simulink model "vipstabilize"  (R2015b)
settings: Solver=FixedStepDiscrete  StartTime=0.0  StopTime=inf  RelTol=1e-3
undefined symbols (not defined in the file or in its folder): gray
libraries: visiontextngfix x3, visiongeotforms x2, visionsinks x2, dspvision x1, vipmisc x1, visionanalysis x1
Description:
  | Image stabilization demo.
settings Model: Tag="0  0  0  0  0  1"  FPTRunName=Active  ExtModeAutoUpdateStatusClock=off  Creator=The MathWorks, Inc.  LastModifiedBy=The MathWorks, Inc.
settings DataIOCC: SaveFormat=Array  SaveOutput=off  SaveTime=off  SignalLoggingName=logsOut
settings OptimizationCC: ExpressionDepthLimit=2147483647  InitFltsAndDblsToZero=on  BufferReusableBoundary=off
settings DebuggingCC: UnderspecifiedInitializationDetection=Classic  MergeDetectMultiDrivingBlocksExec=none  CheckExecutionContextPreStartOutputMsg=on  CheckExecutionContextRuntimeOutputMsg=on  SignalResolutionControl=TryResolveAllWithWarning  InheritedTsInSrcMsg=none  MultiTaskDSMMsg=warning  MultiTaskCondExecSysMsg=none  FcnCallInpInsideContextMsg=UseLocalSettings  BusObjectLabelMismatch=none  StateNameClashWarn=warning  StrictBusMsg=None
settings HardwareCC: ProdBitPerPointer=32  ProdLargestAtomicFloat=None  ProdIntDivRoundTo=Undefined  ProdEndianess=Unspecified  ProdWordSize=32  ProdHWDeviceType=Specified  TargetBitPerLong=64  TargetBitPerPointer=64  TargetLongLongMode=on  TargetIntDivRoundTo=Zero  TargetEndianess=LittleEndian  TargetWordSize=64  TargetHWDeviceType=Generic->MATLAB Host Computer  ProdEqTarget=off
settings ModelReferenceCC: UpdateModelReferenceTargets=IfOutOfDate
settings GRTTargetCC: TargetFcnLib=ansi_tfl_tmw_new.mat  GeneratePreprocessorConditionals=Disable all  CombineOutputUpdateFcns=off  GRTInterface=on
settings ConfigComp: CovModelRefEnable=Off

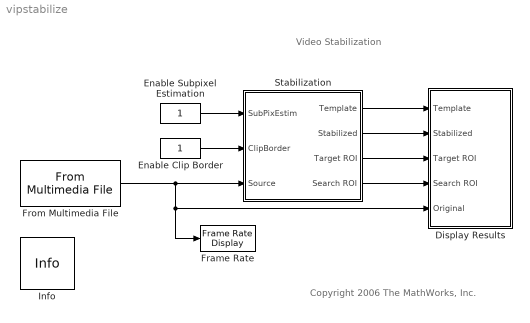
== system vipstabilize ==
  note: Video Stabilization
  note: Copyright 2006 The MathWorks, Inc.
  Display Results : Subsystem
  Enable Clip Border : Constant  VectorParams1D=off  OutDataTypeStr=boolean
  Enable Subpixel Estimation : Constant  VectorParams1D=off  OutDataTypeStr=boolean
  Frame Rate : visionsinks/Frame Rate Display  UpdateRate=10
  From Multimedia File : dspvision/From Multimedia File  inputFilename=shaky_car.avi  loop=on  numPlays=inf  outputStreams=Video only  videoDataType=single  audioDataType=int16  inheritSampleTime=on  userDefinedSampleTime=1/30  noAudioOutput=off  isIntensityVideo=off  fourcc=Intensity  colorVideoFormat=Separate color signals  outputEOF=off  dataOrg=Column-major  audioFrameSize=1024  computeAudioFrameSize=off  outSamplingMode=Frame based
  Info : vipmisc/Info  SystemSampleTime=-1
  Stabilization : Subsystem  mask(Stabilization){template_orig=[109 100], template_size=[18 22], search_border=[10 15]}
      mask prompts: template_orig "Upper left corner of the template [x y]:"; template_size "Template size [height width]:"; search_border "Search border [num_rows num_cols]:"
      mask help:
      | Remove motion from the input video signal.
      |
      | Use Upper left corner of template and Template size parameters to define the location and size of the target on the first frame of the input video.  Use Search border to define size of the search region around the target.
      |
      | Note:  You can right-click on Stabilization subsystem and select "Look Under Mask" to explore the design of the underlying algorithm.
      mask init:
      | pos.template_orig = fliplr(template_orig); % Use R,C internally
      | pos.template_size = template_size;
      | pos.search_border = search_border;
      | pos.template_center = floor((template_size-1)/2);
      | pos.template_center_pos = pos.template_orig + ...
      |     pos.template_center - 1;
      mask Help: Demo subsystem in support of the Video Stabilization demo.  You can right-click on Stabilization subsystem and select "Look Under Mask" to explore the design of the underlying algorithm.
  wires:
  Stabilization/1(Template) -> Display Results/1(Template)
  From Multimedia File/1 -> Display Results/5(Original), Frame Rate/1, Stabilization/3(Source)
  Stabilization/2(Stabilized) -> Display Results/2(Stabilized)
  Enable Subpixel Estimation/1 -> Stabilization/1(SubPixEstim)
  Stabilization/3(Target ROI) -> Display Results/3(Target ROI)
  Stabilization/4(Search ROI) -> Display Results/4(Search ROI)
  Enable Clip Border/1 -> Stabilization/2(ClipBorder)

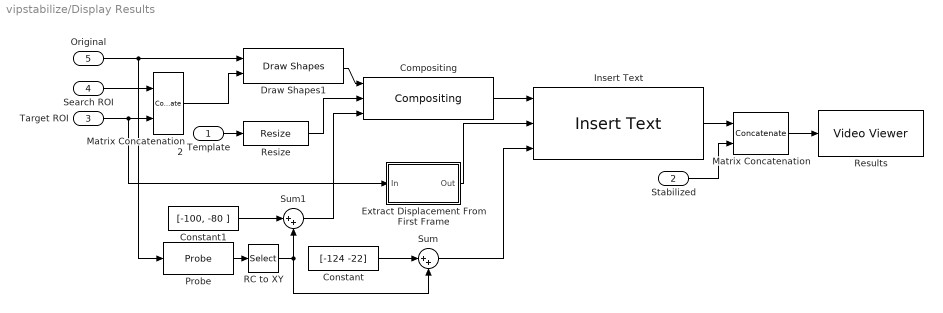
== system vipstabilize/Display Results ==
  Template : Inport
  Stabilized : Inport  Port=2
  Target ROI : Inport  Port=3
  Search ROI : Inport  Port=4
  Original : Inport  Port=5
  Compositing : visiontextngfix/Compositing  operation=Binary mask  bFacSrc=Specify via dialog  mFacSrc=Specify via dialog  bFactor=1  mFactor=1  source=Input port  coordinates=[160 220]  prodOutputMode=Binary point scaling  prodOutputWordLength=32  prodOutputFracLength=10  roundingMode=Floor  overflowMode=off
  Constant : Constant  Value=[-124 -22]
  Constant1 : Constant  Value=[-100, -80 ]
  Draw Shapes1 : visiontextngfix/Draw Shapes  shape=Rectangles  fill=off  lineWidth=1  fillClrSource=Specify via dialog  display=White  intensity=200  color=[200 255 100]  opacity=0.6  viewport=Entire image  antialiasing=off  inType=Intensity  imagePorts=One multidimensional signal  prodOutputMode=Binary point scaling  prodOutputWordLength=32  prodOutputFracLength=14  memoryMode=Specify word length  memoryWordLength=16  memoryFracLength=15  roundingMode=Floor  overflowMode=off
  Extract Displacement From First Frame : Subsystem
  Insert Text : visiontextngfix/Insert Text  inputType=Obsolete  theText='(%+05.1f,%+05.1f)'  getTextLocFrom=Input port  textLoc=[218 196]  getTextColorFrom=Specify via dialog  textColor=1  getTextIntensityFrom=Specify via dialog  textIntensity=1  getTextOpacityFrom=Specify via dialog  textOpacity=1.0  dummyVar2=0  dummyVar3=0  dummyVar4=0  imagePorts=One multidimensional signal  isInputTransposed=off  fontFace=LucidaTypewriterRegular  dummyVar1=0  blockFontSize=14  antiAliased=on
  Matrix Concatenation : Concatenate  Mode=Multidimensional array  ConcatenateDimension=2
  Matrix Concatenation2 : Concatenate  Mode=Multidimensional array
  Probe : Probe  ProbeWidth=off  ProbeSampleTime=off  ProbeComplexSignal=off  ProbeSignalDimensions=on
  RC to XY : Selector  IndexOptions=Index vector (dialog)  Indices=[2 1]  OutputSizes=1
  Resize : visiongeotforms/Resize  specify=Output size as a percentage of input size  rfactor=300  outCols=25  outRows=25  outRowsCols=[25 35]  interp_method=Bilinear  antialias=on  useROI=off  roiFlag=off  prodOutputMode=Binary point scaling  prodOutputWordLength=32  prodOutputFracLength=10  roundingMode=Nearest  overflowMode=on
  Results : visionsinks/Video Viewer  inputType=Obsolete7b  imagePorts=One multidimensional signal  useColorMap=off  colormapValue=gray(256)  specRange=off  minInputVal=0  maxInputVal=255  FigPos=[83 372 640 262]  AxisZoom=on  trueSizedOnce=on  OpenAtMdlStart=on  DefaultConfigurationName=vipscopes.VideoViewerScopeCfg
  Sum : Sum  Inputs=|++
  Sum1 : Sum  Inputs=|++
  wires:
  Stabilized/1 -> Matrix Concatenation/2
  Extract Displacement From First Frame/1(Out) -> Insert Text/2
  Draw Shapes1/1 -> Compositing/1
  Matrix Concatenation2/1 -> Draw Shapes1/2
  Search ROI/1 -> Matrix Concatenation2/1
  Target ROI/1 -> Matrix Concatenation2/2, Extract Displacement From First Frame/1(In)
  Original/1 -> Draw Shapes1/1, Probe/1
  Matrix Concatenation/1 -> Results/1
  Compositing/1 -> Insert Text/1
  Insert Text/1 -> Matrix Concatenation/1
  Resize/1 -> Compositing/2
  Constant1/1 -> Sum1/1
  Sum1/1 -> Compositing/3
  Probe/1 -> RC to XY/1
  Sum/1 -> Insert Text/3
  Constant/1 -> Sum/1
  Template/1 -> Resize/1
  RC to XY/1 -> Sum1/2, Sum/2

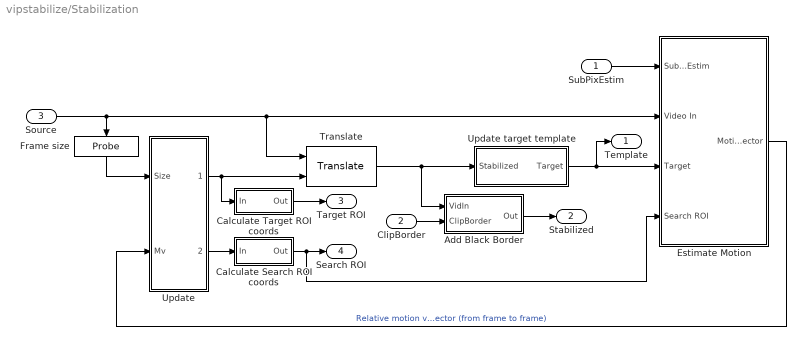
== system vipstabilize/Stabilization ==
  SubPixEstim : Inport
  ClipBorder : Inport  Port=2
  Source : Inport  Port=3
  Add Black Border : Subsystem
  Calculate Search ROI coords : Subsystem
  Calculate Target ROI coords : Subsystem
  Estimate Motion : Subsystem
  Frame size : Probe  ProbeWidth=off  ProbeSampleTime=off  ProbeComplexSignal=off  ProbeSignalDimensions=on  ProbeDimensionsDataType=Same as input
  Translate : visiongeotforms/Translate  outSizeT=Same as input image  src_trans=Input port  translation="[1.5  2.3]"  maxOffset=[8 10]  fillVal=0  interpMethod=Bilinear  firstCoeffMode=Binary point scaling  firstCoeffWordLength=16  firstCoeffFracLength=6  prodOutputMode=Binary point scaling  prodOutputWordLength=16  prodOutputFracLength=10  roundingMode=Floor  overflowMode=off
  Update : Subsystem
  Update target template : Subsystem
  Template : Outport
  Stabilized : Outport  Port=2
  Target ROI : Outport  Port=3
  Search ROI : Outport  Port=4
  wires:
  ClipBorder/1 -> Add Black Border/2(ClipBorder)
  Add Black Border/1(Out) -> Stabilized/1
  Calculate Search ROI coords/1(Out) -> Search ROI/1, Estimate Motion/4(Search ROI)
  Calculate Target ROI coords/1(Out) -> Target ROI/1
  SubPixEstim/1 -> Estimate Motion/1(SubPixEstim)
  Update/1(Offset) -> Calculate Target ROI coords/1(In), Translate/2
  Update/2(Location) -> Calculate Search ROI coords/1(In)
  Update target template/1(Target) -> Template/1, Estimate Motion/3(Target)
  Source/1 -> Translate/1, Estimate Motion/2(Video In), Frame size/1
  Translate/1 -> Add Black Border/1(VidIn), Update target template/1(Stabilized)
  Estimate Motion/1(Motion Vector) -> Update/2(Mv)  "Relative motion vector (from frame to frame)"
  Frame size/1 -> Update/1(Size)

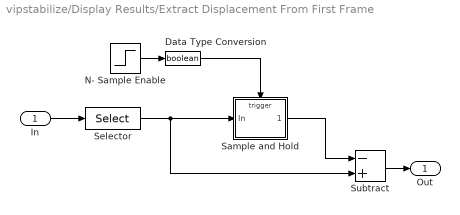
== system vipstabilize/Display Results/Extract Displacement From First Frame ==
  In : Inport
  Data Type Conversion : DataTypeConversion  OutDataTypeStr=boolean
  N- Sample Enable : Step  Time=0
  Sample and Hold : Subsystem  TreatAsAtomicUnit=on  mask{initCond=0}
      mask prompts: initCond "Initial Condition"
  Selector : Selector  NumberOfDimensions=2  InputPortWidth=3  IndexOptions=Index vector (dialog),Index vector (dialog)  Indices=1,[1 2]  OutputSizes=1,1
  Subtract : Sum  Inputs=-+
  Out : Outport
  wires:
  Data Type Conversion/1 -> Sample and Hold/Trigger
  In/1 -> Selector/1
  Selector/1 -> Subtract/2, Sample and Hold/1(In)
  Subtract/1 -> Out/1
  Sample and Hold/1(" ") -> Subtract/1
  N- Sample Enable/1 -> Data Type Conversion/1

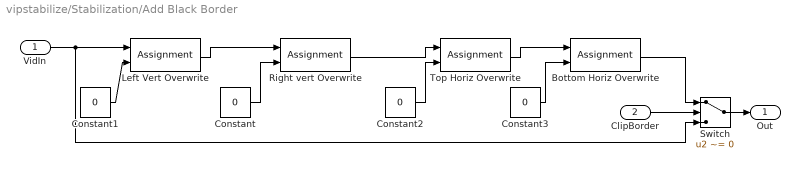
== system vipstabilize/Stabilization/Add Black Border ==
  VidIn : Inport
  ClipBorder : Inport  Port=2
  Bottom Horiz Overwrite : Assignment  NumberOfDimensions=2  IndexOptions=Index vector (dialog),Assign all  Indices=[240-(pos.search_border(2)+4):240],[320-(pos.search_border(2)+4):320]  OutputSizes=1,1
  Constant{,1..3} (4 alike) : Constant  Value=0  OutDataTypeStr=single
  Left Vert Overwrite : Assignment  NumberOfDimensions=2  IndexOptions=Assign all,Index vector (dialog)  Indices=1:end,1:(pos.search_border(2)+4)  OutputSizes=1,1
  Right vert Overwrite : Assignment  NumberOfDimensions=2  IndexOptions=Assign all,Index vector (dialog)  Indices=1:end,[320-(pos.search_border(2)+4):320]  OutputSizes=1,1
  Switch : Switch  Criteria=u2 ~= 0  ZeroCross=off
  Top Horiz Overwrite : Assignment  NumberOfDimensions=2  IndexOptions=Index vector (dialog),Assign all  Indices=[1:pos.search_border(1)+4],[320-(pos.search_border(2)+4):320]  OutputSizes=1,1
  Out : Outport
  wires:
  VidIn/1 -> Switch/3, Left Vert Overwrite/1
  Left Vert Overwrite/1 -> Right vert Overwrite/1
  Right vert Overwrite/1 -> Top Horiz Overwrite/1
  Top Horiz Overwrite/1 -> Bottom Horiz Overwrite/1
  ClipBorder/1 -> Switch/2
  Bottom Horiz Overwrite/1 -> Switch/1
  Switch/1 -> Out/1
  Constant/1 -> Right vert Overwrite/2
  Constant1/1 -> Left Vert Overwrite/2
  Constant2/1 -> Top Horiz Overwrite/2
  Constant3/1 -> Bottom Horiz Overwrite/2

== system vipstabilize/Stabilization/Calculate Search ROI coords ==
  In : Inport
  Constant : Constant  Value=fliplr(pos.template_size + 2*pos.search_border)  VectorParams1D=off  OutDataTypeStr=single
  Flip : Selector  NumberOfDimensions=2  IndexOptions=Index vector (dialog),Index vector (dialog)  Indices=1,[2 1]  OutputSizes=1,1
  Matrix Concatenation : Concatenate  Mode=Multidimensional array  ConcatenateDimension=2
  Out : Outport
  wires:
  Matrix Concatenation/1 -> Out/1
  In/1 -> Flip/1
  Constant/1 -> Matrix Concatenation/2
  Flip/1 -> Matrix Concatenation/1

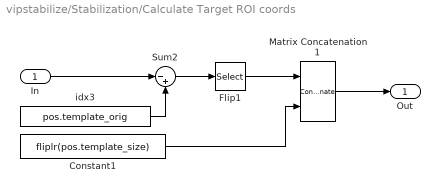
== system vipstabilize/Stabilization/Calculate Target ROI coords ==
  In : Inport
  Constant1 : Constant  Value=fliplr(pos.template_size)  VectorParams1D=off  OutDataTypeStr=single
  Flip1 : Selector  NumberOfDimensions=2  IndexOptions=Index vector (dialog),Index vector (dialog)  Indices=1,[2 1]  OutputSizes=1,1
  Matrix Concatenation1 : Concatenate  Mode=Multidimensional array  ConcatenateDimension=2
  Sum2 : Sum  Inputs=|-+
  idx3 : Constant  Value=pos.template_orig  VectorParams1D=off  OutDataTypeStr=single
  Out : Outport
  wires:
  Matrix Concatenation1/1 -> Out/1
  idx3/1 -> Sum2/2
  Sum2/1 -> Flip1/1
  Constant1/1 -> Matrix Concatenation1/2
  Flip1/1 -> Matrix Concatenation1/1
  In/1 -> Sum2/1

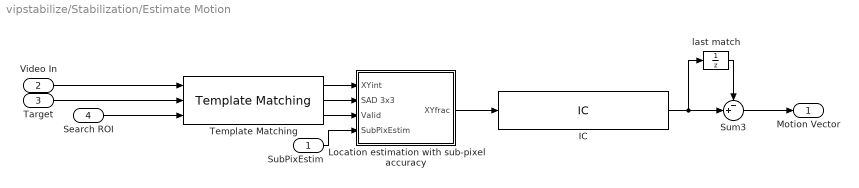
== system vipstabilize/Stabilization/Estimate Motion ==
  SubPixEstim : Inport
  Video In : Inport  Port=2
  Target : Inport  Port=3
  Search ROI : Inport  Port=4
  IC : InitialCondition  Value=fliplr(pos.template_center_pos)
  Location estimation with sub-pixel accuracy : Subsystem
  Sum3 : Sum  Inputs=-+|
  Template Matching : visionanalysis/Template Matching  metric=Sum of absolute differences  output=Best match location  method=Exhaustive  nMetric=on  nSize=3  roi=on  roiValid=off  accumMode=Binary point scaling  accumWordLength=32  accumFracLength=0  prodOutputMode=Binary point scaling  prodOutputWordLength=32  prodOutputFracLength=0  roundingMode=Floor  overflowMode=off
  last match : UnitDelay  InitialCondition=fliplr(pos.template_center_pos)  SampleTime=-1
  Motion Vector : Outport
  wires:
  IC/1 -> last match/1, Sum3/2
  last match/1 -> Sum3/1
  Location estimation with sub-pixel accuracy/1(XYfrac) -> IC/1
  SubPixEstim/1 -> Location estimation with sub-pixel accuracy/4(SubPixEstim)
  Search ROI/1 -> Template Matching/3
  Sum3/1 -> Motion Vector/1
  Target/1 -> Template Matching/2
  Template Matching/1 -> Location estimation with sub-pixel accuracy/1(XYint)
  Template Matching/2 -> Location estimation with sub-pixel accuracy/2(SAD 3x3)
  Template Matching/3 -> Location estimation with sub-pixel accuracy/3(Valid)
  Video In/1 -> Template Matching/1

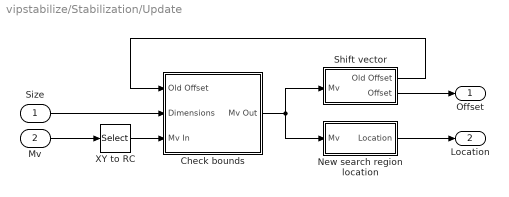
== system vipstabilize/Stabilization/Update ==
  Size : Inport
  Mv : Inport  Port=2
  Check bounds : Subsystem
  New search region location : Subsystem
  Shift vector : Subsystem
  XY to RC : Selector  NumberOfDimensions=2  IndexOptions=Index vector (dialog),Index vector (dialog)  Indices=1,[2 1]  OutputSizes=1,1
  Offset : Outport
  Location : Outport  Port=2
  wires:
  Shift vector/1(Old Offset) -> Check bounds/1(Old Offset)
  Mv/1 -> XY to RC/1
  New search region location/1(Location) -> Location/1
  Shift vector/2(Offset) -> Offset/1
  Size/1 -> Check bounds/2(Dimensions)
  Check bounds/1(Mv Out) -> Shift vector/1(Mv), New search region location/1(Mv)
  XY to RC/1 -> Check bounds/3(Mv In)

== system vipstabilize/Stabilization/Update target template ==
  note: cut out new template
  Stabilized : Inport
  Delay : UnitDelay  SampleTime=-1
  Selector : Selector  NumberOfDimensions=2  InputPortWidth=3  IndexOptions=Index vector (dialog),Index vector (dialog)  Indices=pos.template_orig(1)-1 : pos.template_orig(1)+pos.template_size(1)-2,pos.template_orig(2)-1 : pos.template_orig(2)+pos.template_size(2)-2  OutputSizes=1,1
  Target : Outport
  wires:
  Delay/1 -> Target/1
  Stabilized/1 -> Selector/1
  Selector/1 -> Delay/1

== system vipstabilize/Display Results/Extract Displacement From First Frame/Sample and Hold ==
  In : Inport
  Trigger : TriggerPort  ZeroCross=off
  " " : Outport  InitialOutput=initCond
  wires:
  In/1 -> " "/1

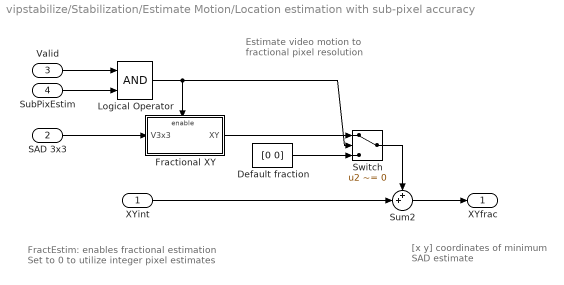
== system vipstabilize/Stabilization/Estimate Motion/Location estimation with sub-pixel accuracy ==
  note: [x y] coordinates of
      | minimum SAD estimate
  note: FractEstim: enables fractional estimation
      | Set to 0 to utilize integer pixel estimates
  note: Estimate video motion to
      | fractional pixel resolution
  XYint : Inport
  SAD 3x3 : Inport  Port=2
  Valid : Inport  Port=3
  SubPixEstim : Inport  Port=4
  Default fraction : Constant  Value=[0 0]  VectorParams1D=off  OutDataTypeStr=Inherit: Inherit via back propagation
  Fractional XY : Subsystem
  Logical Operator : Logic  AllPortsSameDT=off  OutDataTypeStr=boolean
  Sum2 : Sum  Inputs=++|  OutDataTypeStr=single
  Switch : Switch  Criteria=u2 ~= 0
  XYfrac : Outport
  wires:
  SubPixEstim/1 -> Logical Operator/2
  XYint/1 -> Sum2/2
  Fractional XY/1(XY) -> Switch/1
  Switch/1 -> Sum2/1
  Default fraction/1 -> Switch/3
  Sum2/1 -> XYfrac/1
  SAD 3x3/1 -> Fractional XY/1(V3x3)
  Logical Operator/1 -> Fractional XY/Enable, Switch/2
  Valid/1 -> Logical Operator/1

== system vipstabilize/Stabilization/Update/Check bounds ==
  Old Offset : Inport
  Dimensions : Inport  Port=2
  Mv In : Inport  Port=3
  Bounds Test : Subsystem
  Constant : Constant  Value=0  OutDataTypeStr=Inherit: Inherit via back propagation
  Switch : Switch  Criteria=u2 ~= 0  ZeroCross=off
  Mv Out : Outport
  wires:
  Mv In/1 -> Switch/1, Bounds Test/1(new_rel)  "D_i"
  Switch/1 -> Mv Out/1
  Dimensions/1 -> Bounds Test/3(dim)
  Constant/1 -> Switch/3
  Bounds Test/1(inbounds) -> Switch/2
  Old Offset/1 -> Bounds Test/2(old_abs)

== system vipstabilize/Stabilization/Update/New search region location ==
  note: This loop accumulates relative motion vector shifts
  note: Predict new search region location
  Mv : Inport
  Sum2 : Sum  Inputs=++|  OutDataTypeStr=single
  Svi : UnitDelay  InitialCondition=pos.template_orig - pos.search_border - 1  SampleTime=-1
  Location : Outport
  wires:
  Mv/1 -> Sum2/2
  Sum2/1 -> Svi/1
  Svi/1 -> Location/1, Sum2/1  "Upper left corner of the search region"

== system vipstabilize/Stabilization/Update/Shift vector ==
  note: this loop keeps track of the absolute shift of the target
  Mv : Inport
  Sum4 : Sum  Inputs=+-|
  Tvi : UnitDelay  SampleTime=-1
  Old Offset : Outport
  Offset : Outport  Port=2
  wires:
  Mv/1 -> Sum4/2
  Tvi/1 -> Old Offset/1, Sum4/1
  Sum4/1 -> Offset/1, Tvi/1

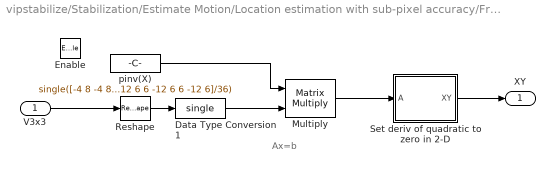
== system vipstabilize/Stabilization/Estimate Motion/Location estimation with sub-pixel accuracy/Fractional XY ==
  note: Ax=b
  V3x3 : Inport
  Enable : EnablePort  StatesWhenEnabling=reset  PropagateVarSize=During execution  ZeroCross=off
  Data Type Conversion1 : DataTypeConversion  OutDataTypeStr=single
  Multiply : Product  Inputs=**  Multiplication=Matrix(*)
  Reshape : Reshape  OutputDimensionality=Column vector (2-D)
  Set deriv of quadratic to zero in 2-D : Subsystem
  pinv(X) : Constant  Value=single([-4 8 -4 8 20 8 -4 8 -4;-6 -6 -6 0 0 0 6 6 6;-6 0 6 -6 0 6 -6 0 6;9 0 -9 0 0 0 -9 0 9;6 6 6 -12 -12 -12 6 6 6;6 -12 6 6 -12 6 6 -12 6]/36)  VectorParams1D=off  OutDataTypeStr=single
  XY : Outport
  wires:
  pinv(X)/1 -> Multiply/1
  Reshape/1 -> Data Type Conversion1/1
  Multiply/1 -> Set deriv of quadratic to zero in 2-D/1(A)
  V3x3/1 -> Reshape/1
  Set deriv of quadratic to zero in 2-D/1(XY) -> XY/1
  Data Type Conversion1/1 -> Multiply/2

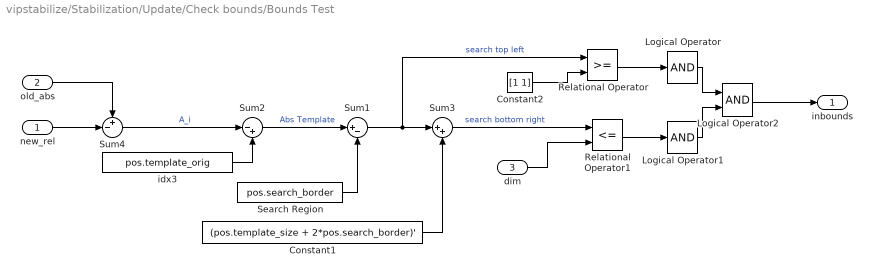
== system vipstabilize/Stabilization/Update/Check bounds/Bounds Test ==
  new_rel : Inport
  old_abs : Inport  Port=2
  dim : Inport  Port=3
  Constant1 : Constant  Value=(pos.template_size + 2*pos.search_border)'  OutDataTypeStr=Inherit: Inherit via back propagation
  Constant2 : Constant  Value=[1 1]  OutDataTypeStr=Inherit: Inherit via back propagation
  Logical Operator : Logic  Inputs=1  AllPortsSameDT=off  OutDataTypeStr=boolean
  Logical Operator1 : Logic  Inputs=1  AllPortsSameDT=off  OutDataTypeStr=boolean
  Logical Operator2 : Logic  AllPortsSameDT=off  OutDataTypeStr=boolean
  Relational Operator : RelationalOperator  OutDataTypeStr=boolean
  Relational Operator1 : RelationalOperator  Operator=<=  OutDataTypeStr=boolean
  Search Region : Constant  Value=pos.search_border  OutDataTypeStr=Inherit: Inherit via back propagation
  Sum1 : Sum  Inputs=|+-  OutDataTypeStr=Inherit: Inherit via back propagation
  Sum2 : Sum  Inputs=|-+  OutDataTypeStr=Inherit: Inherit via back propagation
  Sum3 : Sum  Inputs=|++  OutDataTypeStr=Inherit: Inherit via back propagation
  Sum4 : Sum  Inputs=+-|  OutDataTypeStr=Inherit: Inherit via back propagation
  idx3 : Constant  Value=pos.template_orig  OutDataTypeStr=Inherit: Inherit via back propagation
  inbounds : Outport
  wires:
  Logical Operator1/1 -> Logical Operator2/2
  Logical Operator/1 -> Logical Operator2/1
  Relational Operator/1 -> Logical Operator/1
  Relational Operator1/1 -> Logical Operator1/1
  dim/1 -> Relational Operator1/2
  Sum3/1 -> Relational Operator1/1  "search bottom right"
  Constant2/1 -> Relational Operator/2
  Constant1/1 -> Sum3/2
  Sum1/1 -> Relational Operator/1, Sum3/1  "search top left"
  Search Region/1 -> Sum1/2
  Sum2/1 -> Sum1/1  "Abs Template"
  idx3/1 -> Sum2/2
  Sum4/1 -> Sum2/1  "A_i"
  old_abs/1 -> Sum4/1
  new_rel/1 -> Sum4/2
  Logical Operator2/1 -> inbounds/1

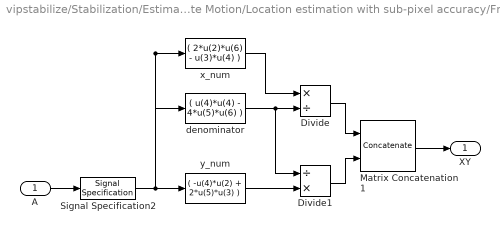
== system vipstabilize/Stabilization/Estimate Motion/Location estimation with sub-pixel accuracy/Fractional XY/Set deriv of quadratic to zero in 2-D ==
  A : Inport
  Divide : Product  Inputs=*/
  Divide1 : Product  Inputs=/*
  Matrix Concatenation1 : Concatenate  Mode=Multidimensional array  ConcatenateDimension=2
  Signal Specification2 : SignalSpecification  Dimensions=[6 1]
  denominator : Fcn  Expr=( u(4)*u(4) - 4*u(5)*u(6) )
  x_num : Fcn  Expr=( 2*u(2)*u(6) - u(3)*u(4) )
  y_num : Fcn  Expr=( -u(4)*u(2) + 2*u(5)*u(3) )
  XY : Outport
  wires:
  A/1 -> Signal Specification2/1
  Signal Specification2/1 -> x_num/1, denominator/1, y_num/1
  Matrix Concatenation1/1 -> XY/1
  x_num/1 -> Divide/1
  denominator/1 -> Divide/2, Divide1/1
  Divide/1 -> Matrix Concatenation1/1
  Divide1/1 -> Matrix Concatenation1/2
  y_num/1 -> Divide1/2
